simulink library "linearPathDomainPlnt_cl"  (R2018b)
settings: Solver=VariableStepAuto  StartTime=0.0  StopTime=10.0  RelTol=1e-3
values from neighbouring files (symbols this model uses):
  initialHeading_deg = 0    [linearPathDomainPlnt_ts.m]
  initialSpeed_mPs = 0    [linearPathDomainPlnt_ts.m]
  initialXPosition_m = 0    [linearPathDomainPlnt_ts.m]
  initialYPosition_m = 0    [linearPathDomainPlnt_ts.m]
libraries: linearPathDomainPlnt_ul x1
settings Model: Creator=mcobb  LastModifiedBy=mcobb
settings DebuggingCC: LibraryContextMissingDiagnostic=none
settings SFSimCC: SimUseLocalCustomCode=off
settings RTWCC: RTWUseLocalCustomCode=off

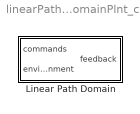
== system linearPathDomainPlnt_cl ==
  Linear Path Domain : Subsystem  VariantControl=VSS_LINEARPATHDOMAIN_PLNT

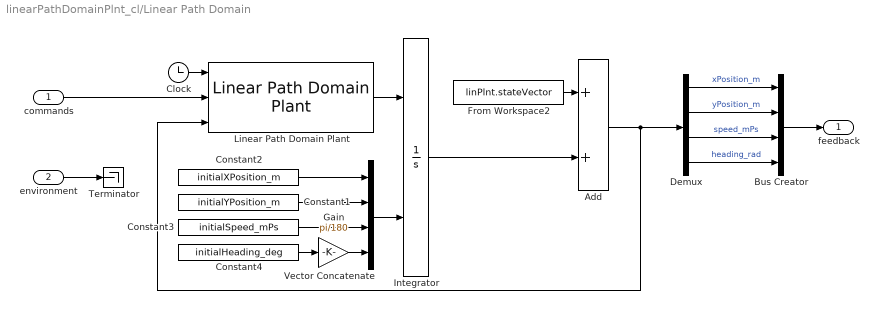
== system linearPathDomainPlnt_cl/Linear Path Domain ==
  commands : Inport
  environment : Inport  Port=2
  Add : Sum
  Bus Creator : BusCreator  Inputs=4
  Clock : Clock
  Constant1 : Constant  Value=initialYPosition_m
  Constant2 : Constant  Value=initialXPosition_m
  Constant3 : Constant  Value=initialSpeed_mPs
  Constant4 : Constant  Value=initialHeading_deg
  Demux : Demux
  From Workspace2 : FromWorkspace  VariableName=linPlnt.stateVector  SampleTime=0
  Gain : Gain  Gain=pi/180
  Integrator : Integrator  InitialConditionSource=external
  Linear Path Domain Plant : linearPathDomainPlnt_ul/Linear Path Domain Plant  SystemSampleTime=-1
  Terminator : Terminator
  Vector Concatenate : Concatenate  NumInputs=4
  feedback : Outport
  wires:
  Vector Concatenate/1 -> Integrator/2
  Constant1/1 -> Vector Concatenate/2
  Linear Path Domain Plant/1 -> Integrator/1
  Constant3/1 -> Vector Concatenate/3
  Constant4/1 -> Gain/1
  Constant2/1 -> Vector Concatenate/1
  Gain/1 -> Vector Concatenate/4
  Demux/1 -> Bus Creator/1  "xPosition_m"
  Demux/2 -> Bus Creator/2  "yPosition_m"
  Demux/3 -> Bus Creator/3  "speed_mPs"
  Demux/4 -> Bus Creator/4  "heading_rad"
  Bus Creator/1 -> feedback/1
  commands/1 -> Linear Path Domain Plant/2
  Add/1 -> Demux/1, Linear Path Domain Plant/3
  Integrator/1 -> Add/2
  Clock/1 -> Linear Path Domain Plant/1
  From Workspace2/1 -> Add/1
  environment/1 -> Terminator/1
